simulink model "StSys_Strt"  (R2016b)
settings: configuration reference "CodeGenConfigSet" (kept outside this file)
values from neighbouring files (symbols this model uses):
  StSys_nStrtCutOut_MAP = Calibration.Parameter    [init_StSys_Strt.m]
  StSys_nStrtCutOut_MAPX = Calibration.Parameter    [init_StSys_Strt.m]
  StSys_nStrtCutOut_MAPY = Calibration.Parameter    [init_StSys_Strt.m]
  StSys_tiStrtCutOut_C = Calibration.Parameter    [init_StSys_Strt.m]
undefined symbols (not defined in the file or in its folder): EngState_conv, StSys_Strt_DT, StSys_StrtState_conv
libraries: CXLib x2
settings Model: Creator=Colin  LastModifiedBy=Administrator
settings ConfigSetRef: SourceLocation=Base Workspace

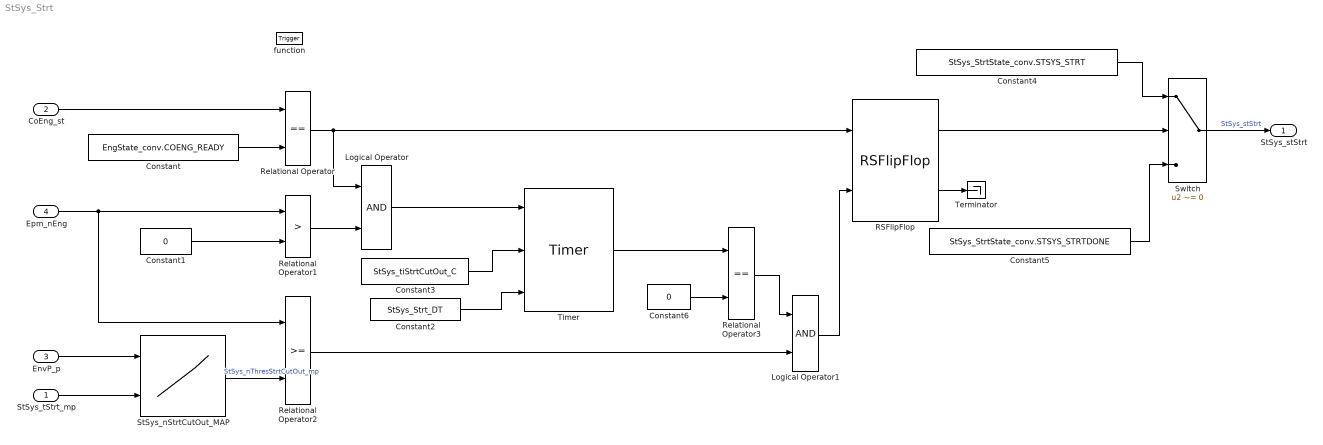
== system StSys_Strt ==
  StSys_tStrt_mp : Inport  Tag=deg  Description=engine temperature for starting system  OutMin=-50  OutMax=150  OutDataTypeStr=Temp_deg
  CoEng_st : Inport  Description=Engine coordinator state  Port=2  OutDataTypeStr=Enum: EngState_conv
  EnvP_p : Inport  Tag=kPa  Description=Barometric pressure  Port=3  OutMin=0  OutMax=3276  OutDataTypeStr=AirPressure_kPa
  Epm_nEng : Inport  Tag=rpm  Description=Engine speed  Port=4  OutMin=0  OutMax=6000  OutDataTypeStr=EngSpeed_rpm
  function : TriggerPort  TriggerType=function-call  VariantControl=Variant
  Constant : Constant  Value=EngState_conv.COENG_READY
  Constant1 : Constant  Value=0  OutDataTypeStr=EngSpeed_rpm
  Constant2 : Constant  Value=StSys_Strt_DT  OutDataTypeStr=EngTime_ms
  Constant3 : Constant  Value=StSys_tiStrtCutOut_C
  Constant4 : Constant  Value=StSys_StrtState_conv.STSYS_STRT
  Constant5 : Constant  Value=StSys_StrtState_conv.STSYS_STRTDONE
  Constant6 : Constant  Value=0  OutDataTypeStr=Inherit: Inherit via back propagation
  Logical Operator : Logic  AllPortsSameDT=off  OutDataTypeStr=boolean
  Logical Operator1 : Logic  AllPortsSameDT=off  OutDataTypeStr=boolean
  RSFlipFlop : CXLib/RSFlipFlop
  Relational Operator : RelationalOperator  Operator===  OutDataTypeStr=boolean  RndMeth=Simplest
  Relational Operator1 : RelationalOperator  Operator=>  OutDataTypeStr=boolean  RndMeth=Simplest
  Relational Operator2 : RelationalOperator  OutDataTypeStr=boolean  RndMeth=Simplest
  Relational Operator3 : RelationalOperator  Operator===  OutDataTypeStr=boolean  RndMeth=Simplest  InputSameDT=on
  StSys_nStrtCutOut_MAP : Lookup_n-D  BreakpointsForDimension1=StSys_nStrtCutOut_MAPY  BreakpointsForDimension2=StSys_nStrtCutOut_MAPX  Table=StSys_nStrtCutOut_MAP  ExtrapMethod=Clip  InternalRulePriority=Speed  OutDataTypeStr=Inherit: Inherit from 'Table data'  RndMeth=Simplest  SaturateOnIntegerOverflow=on
  Switch : Switch  Criteria=u2 ~= 0
  Terminator : Terminator
  Timer : CXLib/Timer
  StSys_stStrt : Outport  Description=state of starting system  OutDataTypeStr=Enum: StSys_StrtState_conv
  wires:
  CoEng_st/1 -> Relational Operator/1
  Constant/1 -> Relational Operator/2
  Epm_nEng/1 -> Relational Operator2/1, Relational Operator1/1
  Constant1/1 -> Relational Operator1/2
  EnvP_p/1 -> StSys_nStrtCutOut_MAP/1
  StSys_tStrt_mp/1 -> StSys_nStrtCutOut_MAP/2
  StSys_nStrtCutOut_MAP/1 -> Relational Operator2/2  "StSys_nThresStrtCutOut_mp"
  Relational Operator/1 -> Logical Operator/1, RSFlipFlop/1
  Relational Operator1/1 -> Logical Operator/2
  Logical Operator/1 -> Timer/1
  Constant2/1 -> Timer/3
  Timer/1 -> Relational Operator3/1
  Relational Operator2/1 -> Logical Operator1/2
  Relational Operator3/1 -> Logical Operator1/1
  Logical Operator1/1 -> RSFlipFlop/2
  Switch/1 -> StSys_stStrt/1  "StSys_stStrt"
  RSFlipFlop/1 -> Switch/2
  RSFlipFlop/2 -> Terminator/1
  Constant4/1 -> Switch/1
  Constant5/1 -> Switch/3
  Constant3/1 -> Timer/2
  Constant6/1 -> Relational Operator3/2
